simulink model "PMSM_Trapezoidal"  (R2013b)
settings: Solver=ode45  StartTime=0.0  StopTime=8  RelTol=1e-3
undefined symbols (not defined in the file): Plot_PMSM
libraries: powerlib x6, simulink x3, powerlib_extras x1
CloseFcn:
  | clear p4 p7 param5 param6 param8 parametres tout visible
settings Model: Creator=Alex  LastModifiedBy=reynaudp
settings OptimizationCC: ExpressionDepthLimit=2147483647
settings DebuggingCC: UnconnectedLineMsg=none  StateNameClashWarn=warning

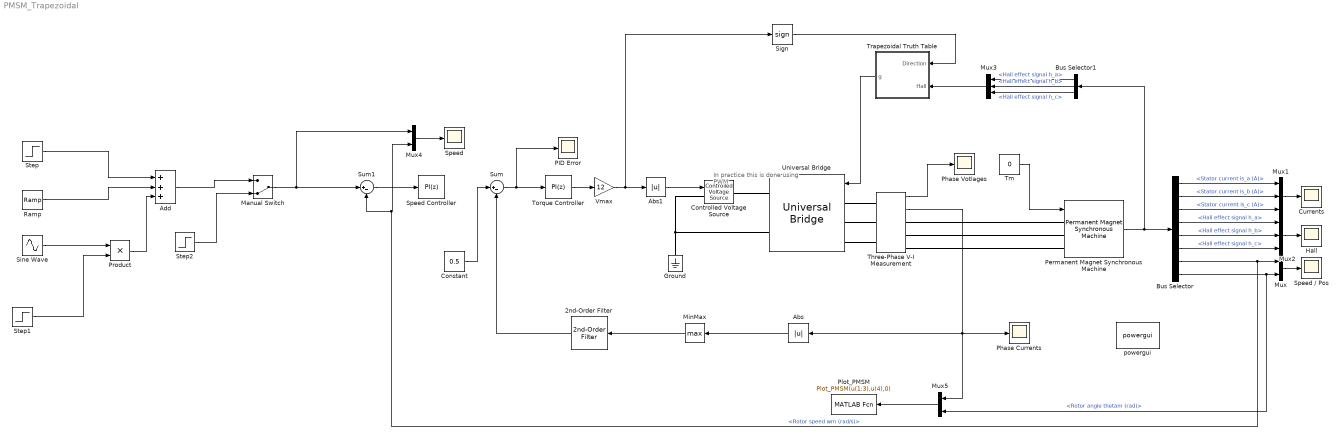
== system PMSM_Trapezoidal ==
  note: In practice this is done using PWM
  2nd-Order Filter : powerlib_extras/Control  Blocks/2nd-Order Filter  FilterType=Lowpass  Fo=300  Zeta=0.707  Initialize=off  Vac_Init=[1 45 60]  Vdc_Init=-0.5  PlotResponse=off  param1=[1 500 1]
  Abs : Abs
  Abs1 : Abs
  Add : Sum  Inputs=+++
  Bus Selector : BusSelector  OutputSignals=Stator current is_a (A),Stator current is_b (A),Stator current is_c (A),Hall effect signal h_a,Hall effect signal h_b,Hall effect signal h_c,Rotor speed wm (rad/s),Rotor angle thetam (rad)
  Bus Selector1 : BusSelector  OutputSignals=Hall effect signal h_a,Hall effect signal h_b,Hall effect signal h_c
  Constant : Constant  Value=0.5
  Controlled Voltage Source : powerlib/Electrical Sources/Controlled Voltage Source  Initialize=on  Source_Type=AC  Amplitude=0  Phase=0  Frequency=0  Measurements=None
  Currents : Scope
      settings: YMin=-1  YMax=1
  Ground : powerlib/Elements/Ground  LConnTagsString=a
  Hall : Scope
      settings: ShowLegends=on  TimeRange=1  YMin=0  YMax=1  SaveName=ScopeData2
  Manual Switch : ManualSwitch  CurrentSetting=0
  MinMax : MinMax  Function=max
  Mux : Mux  Inputs=2
  Mux1 : Mux  Inputs=3
  Mux2 : Mux  Inputs=3
  Mux3 : Mux  Inputs=3
  Mux4 : Mux  Inputs=2
  Mux5 : Mux  Inputs=2
  PID Error : Scope
      settings: YMin=-1  YMax=0.5  SaveName=ScopeData4
  Permanent Magnet Synchronous Machine : powerlib/Machines/Permanent Magnet Synchronous Machine  NbPhases=3  FluxDistribution=Sinusoidal  RotorType=Round  MechanicalLoad=Torque Tm  PresetModel=No  ShowDetailedParameters=on  Resistance=0.6  Inductance=1.4e-3  dqInductances=[8.5e-3,8.5e-3]  La=0.000835  MachineConstant=Voltage Constant (V_peak L-L / krpm)  Flux=0.034064  VoltageCst=6.1785  TorqueCst=0.051096  Flat=120  Mechanical=[1.1e-5,0,1,0.02]  PolePairs=1  InitialConditions=[1,0 0,0]  InitialConditions5ph=[0 0 0 0 0 0]  TsPowergui=0  TsBlock=-1  RefAngle=Aligned with phase A axis (original Park)
  Phase Currents : Scope
      settings: YMin=-4  YMax=4  SaveName=ScopeData5
  Phase Votlages : Scope
      settings: YMin=-0.025  YMax=0.3  SaveName=ScopeData3
  Plot_PMSM : MATLABFcn  MATLABFcn=Plot_PMSM(u(1:3),u(4),0)  OutputDimensions=0  SampleTime=1/100
  Product : Product  RndMeth=Zero
  Ramp : simulink/Sources/Ramp  slope=50  start=2  X0=0
  Sign : Signum
  Sine Wave : Sin  Amplitude=20  Frequency=2*pi  SampleTime=0
  Speed : Scope
      settings: YMin=-10  YMax=140  SaveName=ScopeData6
  Speed / Pos : Scope
      settings: ShowLegends=on  TimeRange=8  YMin=145  YMax=255
  Speed Controller : simulink/Continuous/PID Controller  Controller=PI  TimeDomain=Discrete-time  SampleTime=1/300  IntegratorMethod=Forward Euler  FilterMethod=Forward Euler  Form=Parallel  P=0.05  I=0.1  D=0.1  N=100  InitialConditionSource=internal  InitialConditionForIntegrator=0  InitialConditionForFilter=0  ExternalReset=none  LimitOutput=on  UpperSaturationLimit=20  LowerSaturationLimit=-20  LinearizeAsGain=off  AntiWindupMode=none  Kb=1  TrackingMode=off  Kt=1  PParamMin=[]  PParamMax=[]  IParamMin=[]  IParamMax=[]  DParamMin=[]  DParamMax=[]  NParamMin=[]  NParamMax=[]  KbParamMin=[]  KbParamMax=[]  KtParamMin=[]  KtParamMax=[]  POutMin=[]  POutMax=[]  IOutMin=[]  IOutMax=[]  DOutMin=[]  DOutMax=[]  NOutMin=[]  NOutMax=[]  KbOutMin=[]  KbOutMax=[]  KtOutMin=[]  KtOutMax=[]  IntegratorOutMin=[]  IntegratorOutMax=[]  FilterOutMin=[]  FilterOutMax=[]  SumOutMin=[]  SumOutMax=[]  SumI1OutMin=[]  SumI1OutMax=[]  SumI2OutMin=[]  SumI2OutMax=[]  SumI3OutMin=[]  SumI3OutMax=[]  SumDOutMin=[]  SumDOutMax=[]  SaturationOutMin=[]  SaturationOutMax=[]  IntegratorContinuousStateAttributes=''  IntegratorStateMustResolveToSignalObject=off  IntegratorRTWStateStorageClass=Auto  FilterContinuousStateAttributes=''  FilterStateMustResolveToSignalObject=off  FilterRTWStateStorageClass=Auto
  Step : Step  Time=0.5  Before=-50  After=-80  SampleTime=0
  Step1 : Step  Time=4  SampleTime=0
  Step2 : Step  Time=.1  After=130  SampleTime=0
  Sum : Sum  Inputs=|+-
  Sum1 : Sum  Inputs=|+-
  Three-Phase V-I Measurement : powerlib/Measurements/Three-Phase V-I Measurement  VoltageMeasurement=phase-to-ground  SetLabelV=off  LabelV=Vabc  Vpu=off  VpuLL=off  CurrentMeasurement=yes  SetLabelI=off  LabelI=Iabc  Ipu=off  Pbase=100e6  Vbase=500e3  OutputType=Complex  PhasorSimulation=off  PSBequivalent=0
  Tm : Constant  Value=0
  Torque Controller : simulink/Continuous/PID Controller  Controller=PI  TimeDomain=Discrete-time  SampleTime=1/300  IntegratorMethod=Trapezoidal  FilterMethod=Forward Euler  Form=Parallel  P=0  I=2  D=0  N=100  InitialConditionSource=internal  InitialConditionForIntegrator=0  InitialConditionForFilter=0  ExternalReset=none  LimitOutput=on  UpperSaturationLimit=1  LowerSaturationLimit=-1  LinearizeAsGain=off  AntiWindupMode=none  Kb=1  TrackingMode=off  Kt=1  PParamMin=[]  PParamMax=[]  IParamMin=[]  IParamMax=[]  DParamMin=[]  DParamMax=[]  NParamMin=[]  NParamMax=[]  KbParamMin=[]  KbParamMax=[]  KtParamMin=[]  KtParamMax=[]  POutMin=[]  POutMax=[]  IOutMin=[]  IOutMax=[]  DOutMin=[]  DOutMax=[]  NOutMin=[]  NOutMax=[]  KbOutMin=[]  KbOutMax=[]  KtOutMin=[]  KtOutMax=[]  IntegratorOutMin=[]  IntegratorOutMax=[]  FilterOutMin=[]  FilterOutMax=[]  SumOutMin=[]  SumOutMax=[]  SumI1OutMin=[]  SumI1OutMax=[]  SumI2OutMin=[]  SumI2OutMax=[]  SumI3OutMin=[]  SumI3OutMax=[]  SumDOutMin=[]  SumDOutMax=[]  SaturationOutMin=[]  SaturationOutMax=[]  IntegratorContinuousStateAttributes=''  IntegratorStateMustResolveToSignalObject=off  IntegratorRTWStateStorageClass=Auto  FilterContinuousStateAttributes=''  FilterStateMustResolveToSignalObject=off  FilterRTWStateStorageClass=Auto
  Trapezoidal Truth Table : MATLAB Function  TreatAsAtomicUnit=on  SystemSampleTime=1/300
  Universal Bridge : powerlib/Power Electronics/Universal Bridge  Arms=3  SnubberResistance=1e5  SnubberCapacitance=inf  Device=MOSFET / Diodes  Ron=1e-3  Lon=0  ForwardVoltages="[  0  0  ]"  ForwardVoltage=0  GTOparameters=[ 10e-6 , 20e-6 ]  IGBTparameters=[ 1e-6 , 2e-6 ]  Measurements=None  Measurements_2=None  converterType=Rectifier
  Vmax : Gain  Gain=12
  powergui : powerlib/powergui  Priority=1  SimulationMode=Discrete  SolverType=Tustin  SampleTime=10e-6  frequency=60  SPID=off  DisableSnubberDevices=off  DisableRonSwitches=off  DisableVfSwitches=off  SwTol=0  Interpol=off  DisplayEquations=off  frequencyindice=0  Pbase=100e6  ErrMax=1e-4  Iterations=50  UnitsV=kV  UnitsW=MW  FunctionMessages=off  echomessages=off  HookPort=off  EnableUseOfTLC=off  x0status=blocks  RestoreLinks=warning  ResistiveCurrentMeasurement=off  Frange=[0:2:500]  Ylog=off  Xlog=on  ShowGrid=off  save=off  variable=ZData  ZoomFFT=off  StartTime=0.0  cycles=1  DisplayStyle=1  fundamental=60  FreqAxis=off  MaxFrequency=1000  frequencyindicesteady=1  RmsSteady=1  display=off  Ts=0  methode=off
  wires:
  Bus Selector/1 -> Mux1/1  "<Stator current is_a (A)>"
  Bus Selector/2 -> Mux1/2  "<Stator current is_b (A)>"
  Bus Selector/3 -> Mux1/3  "<Stator current is_c (A)>"
  Bus Selector/8 -> Mux5/2, Mux/2  "<Rotor angle thetam (rad)>"
  Mux1/1 -> Currents/1
  Tm/1 -> Permanent Magnet Synchronous Machine/1
  Permanent Magnet Synchronous Machine/1 -> Bus Selector1/1, Bus Selector/1
  Bus Selector/7 -> Sum1/2, Mux4/2, Mux/1  "<Rotor speed wm (rad/s)>"
  Bus Selector/4 -> Mux2/1  "<Hall effect signal h_a>"
  Bus Selector/5 -> Mux2/2  "<Hall effect signal h_b>"
  Bus Selector/6 -> Mux2/3  "<Hall effect signal h_c>"
  Mux2/1 -> Hall/1
  Sum/1 -> PID Error/1, Torque Controller/1
  Three-Phase V-I Measurement/2 -> Mux5/1, Phase Currents/1, Abs/1
  Abs/1 -> MinMax/1
  Bus Selector1/1 -> Mux3/1  "<Hall effect signal h_a>"
  Bus Selector1/2 -> Mux3/2  "<Hall effect signal h_b>"
  Bus Selector1/3 -> Mux3/3  "<Hall effect signal h_c>"
  Mux3/1 -> Trapezoidal Truth Table/2(Hall)
  Three-Phase V-I Measurement/1 -> Phase Votlages/1
  Torque Controller/1 -> Vmax/1
  Vmax/1 -> Sign/1, Abs1/1
  Trapezoidal Truth Table/1(g) -> Universal Bridge/1
  Sum1/1 -> Speed Controller/1
  Mux/1 -> Speed / Pos/1
  Mux4/1 -> Speed/1
  Step/1 -> Add/1
  Ramp/1 -> Add/2
  Sine Wave/1 -> Product/1
  Step1/1 -> Product/2
  Product/1 -> Add/3
  Sign/1 -> Trapezoidal Truth Table/1(Direction)
  Abs1/1 -> Controlled Voltage Source/1
  Add/1 -> Manual Switch/1
  Manual Switch/1 -> Mux4/1, Sum1/1
  Step2/1 -> Manual Switch/2
  Mux5/1 -> Plot_PMSM/1
  MinMax/1 -> 2nd-Order Filter/1
  Constant/1 -> Sum/1
  2nd-Order Filter/1 -> Sum/2
  connections:
  Three-Phase V-I Measurement/RConn1 -- Permanent Magnet Synchronous Machine/LConn1
  Three-Phase V-I Measurement/RConn2 -- Permanent Magnet Synchronous Machine/LConn2
  Three-Phase V-I Measurement/RConn3 -- Permanent Magnet Synchronous Machine/LConn3
  Controlled Voltage Source/LConn1 -- Ground/LConn1 -- Universal Bridge/RConn2
  Controlled Voltage Source/RConn1 -- Universal Bridge/RConn1
  Universal Bridge/LConn1 -- Three-Phase V-I Measurement/LConn1
  Universal Bridge/LConn2 -- Three-Phase V-I Measurement/LConn2
  Universal Bridge/LConn3 -- Three-Phase V-I Measurement/LConn3

== matlab function PMSM_Trapezoidal/Trapezoidal Truth Table ==
  data: Direction input; g output; Hall input
function g = fcn(Direction,Hall)

g = nan(6,1);
LUP = zeros(2,2,2,6);
if Direction == 1
    LUP(2,2,1,:) = [0 0 1 0 0 1];
    LUP(1,2,1,:) = [0 1 1 0 0 0];
    LUP(1,2,2,:) = [0 1 0 0 1 0];
    LUP(1,1,2,:) = [0 0 0 1 1 0];
    LUP(2,1,2,:) = [1 0 0 1 0 0];
    LUP(2,1,1,:) = [1 0 0 0 0 1];
else
    LUP(2,2,1,:) = [0 0 0 1 1 0];
    LUP(1,2,1,:) = [1 0 0 1 0 0];
    LUP(1,2,2,:) = [1 0 0 0 0 1];
    LUP(1,1,2,:) = [0 0 1 0 0 1];
    LUP(2,1,2,:) = [0 1 1 0 0 0];
    LUP(2,1,1,:) = [0 1 0 0 1 0];
end

g(:) = LUP(Hall(1)+1,Hall(2)+1,Hall(3)+1,:);
